simulink subsystem "compFilter"  (R2026a)
settings: Solver=VariableStepAuto
values from neighbouring files (symbols this model uses):
  navComp = 0.99    [navParams.sldd]
  navControl = 1    [navParams.sldd]
undefined symbols (not defined in the file or in its folder): flightMode
libraries: simulink x1, sharedutil x1
settings Model: Creator=maxhu  LastModifiedBy=maxhu

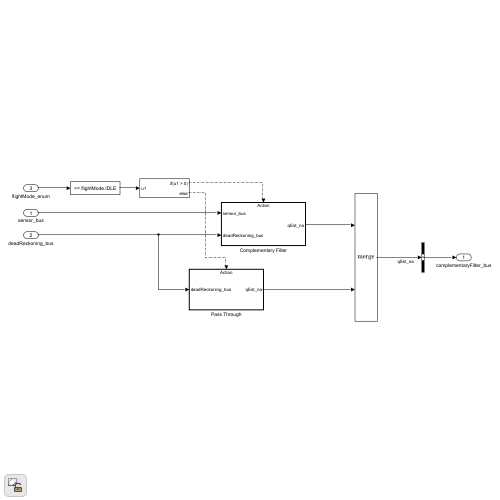
[thumbnail: Simulink's stored preview of the top-level diagram]
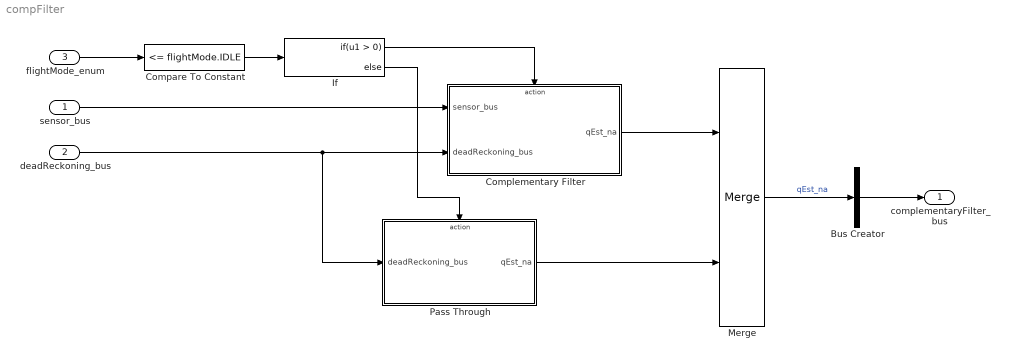
== system compFilter ==
  sensor_bus : Inport
  deadReckoning_bus : Inport  Port=2
  flightMode_enum : Inport  Port=3
  Bus Creator : BusCreator  Inputs=1
  Compare To Constant : simulink/Logic and Bit Operations/Compare To Constant  relop=<=  const=flightMode.IDLE  OutDataTypeStr=boolean
  Complementary Filter : Subsystem  TreatAsAtomicUnit=on
  If : If
  Merge : Merge
  Pass Through : Subsystem  TreatAsAtomicUnit=on
  complementaryFilter_bus : Outport
  wires:
  Merge/1 -> Bus Creator/1  "qEst_na"
  Bus Creator/1 -> complementaryFilter_bus/1
  flightMode_enum/1 -> Compare To Constant/1
  Compare To Constant/1 -> If/1
  If/1 -> Complementary Filter/Action
  If/2 -> Pass Through/Action
  deadReckoning_bus/1 -> Complementary Filter/2(deadReckoning_bus), Pass Through/1(deadReckoning_bus)
  sensor_bus/1 -> Complementary Filter/1(sensor_bus)
  Complementary Filter/1(qEst_na) -> Merge/1
  Pass Through/1(qEst_na) -> Merge/2

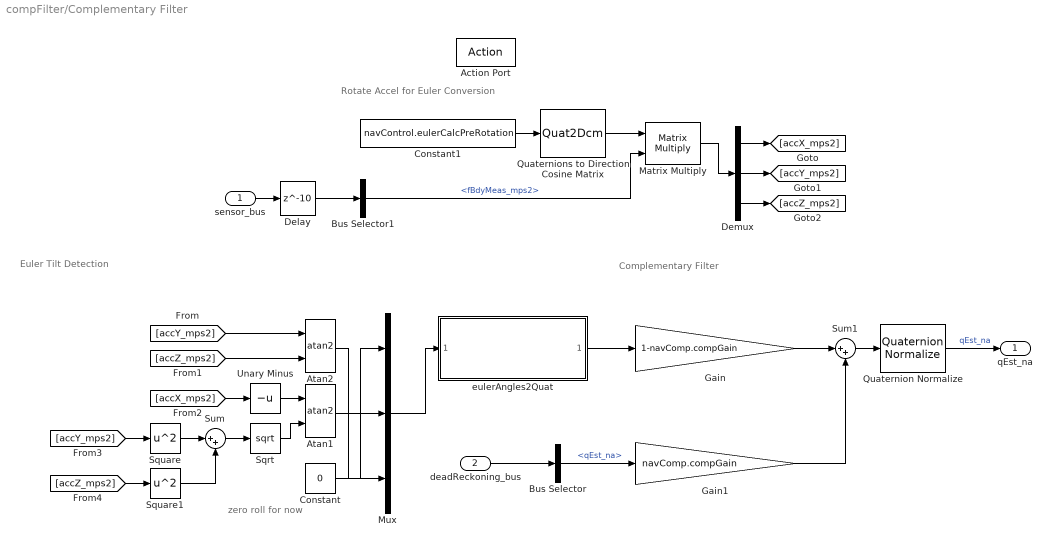
== system compFilter/Complementary Filter ==
  note: Rotate Accel for Euler Conversion
  note: Euler Tilt Detection
  note: Complementary Filter
  note: zero roll for now
  sensor_bus : Inport
  deadReckoning_bus : Inport  Port=2
  Action Port : ActionPort
  Atan1 : Trigonometry  Operator=atan2
  Atan2 : Trigonometry  Operator=atan2
  Bus Selector : BusSelector  OutputSignals=qEst_na
  Bus Selector1 : BusSelector  OutputSignals=fBdyMeas_mps2
  Constant : Constant  Value=0
  Constant1 : Constant  Value=navControl.eulerCalcPreRotation
  Delay : Delay  DelayLength=10
  Demux : Demux  Outputs=3
  Gain : Gain  Gain=1-navComp.compGain
  Gain1 : Gain  Gain=navComp.compGain
  Matrix Multiply : Product  Multiplication=Matrix(*)
  Mux : Mux  Inputs=3
  Quaternion Normalize : sharedutil/Quaternion Normalize  aMode=aMode
  Quaternions to Direction Cosine Matrix : Quat2Dcm
  Sqrt : Sqrt
  Square : Math  Operator=square
  Square1 : Math  Operator=square
  Sum : Sum  Inputs=|++
  Sum1 : Sum  Inputs=|++
  Unary Minus : UnaryMinus
  eulerAngles2Quat : Subsystem  ReferencedSubsystem=eulerAngles2Quat
  qEst_na : Outport
  wires:
  Atan2/1 -> Mux/3
  Constant/1 -> Mux/1
  Quaternion Normalize/1 -> qEst_na/1  "qEst_na"
  Matrix Multiply/1 -> Demux/1
  [accY_mps2] -> Square/1
  Gain1/1 -> Sum1/2
  Bus Selector/1 -> Gain1/1  "<qEst_na>"
  Square/1 -> Sum/1
  Sum/1 -> Sqrt/1
  Atan1/1 -> Mux/2
  eulerAngles2Quat/1 -> Gain/1
  Demux/1 -> [accX_mps2]
  sensor_bus/1 -> Delay/1
  Bus Selector1/1 -> Matrix Multiply/2  "<fBdyMeas_mps2>"
  Square1/1 -> Sum/2
  Gain/1 -> Sum1/1
  Demux/2 -> [accY_mps2]
  Demux/3 -> [accZ_mps2]
  Unary Minus/1 -> Atan1/1
  [accZ_mps2] -> Square1/1
  Sum1/1 -> Quaternion Normalize/1
  Sqrt/1 -> Atan1/2
  Constant1/1 -> Quaternions to Direction Cosine Matrix/1
  deadReckoning_bus/1 -> Bus Selector/1
  Mux/1 -> eulerAngles2Quat/1
  Delay/1 -> Bus Selector1/1
  [accY_mps2] -> Atan2/1
  [accX_mps2] -> Unary Minus/1
  [accZ_mps2] -> Atan2/2
  Quaternions to Direction Cosine Matrix/1 -> Matrix Multiply/1

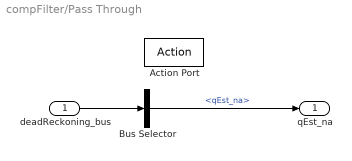
== system compFilter/Pass Through ==
  deadReckoning_bus : Inport
  Action Port : ActionPort
  Bus Selector : BusSelector  OutputSignals=qEst_na
  qEst_na : Outport
  wires:
  Bus Selector/1 -> qEst_na/1  "<qEst_na>"
  deadReckoning_bus/1 -> Bus Selector/1
